simulink model "teste_bar_dados_5_1"  (R2020a)
settings: Solver=VariableStepAuto  StartTime=0.0  StopTime=10.0  RelTol=1e-3
values from neighbouring files (symbols this model uses):
  sample_time = 0.03    [lab3.m]
settings Model: Creator=josem  LastModifiedBy=josem

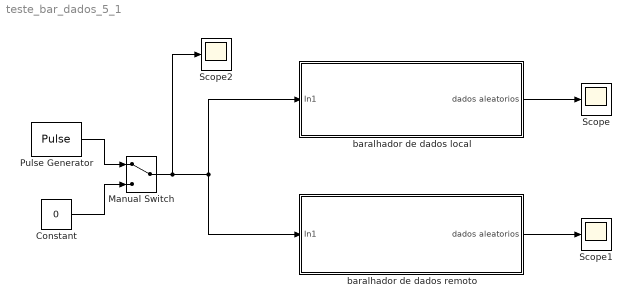
== system teste_bar_dados_5_1 ==
  Constant : Constant  Value=0  SampleTime=sample_time
  Manual Switch : ManualSwitch
  Pulse Generator : DiscretePulseGenerator  Period=10  PulseWidth=5  SampleTime=sample_time
  Scope : Scope
  Scope1 : Scope
  Scope2 : Scope
  baralhador de dados local : Subsystem
  baralhador de dados remoto : Subsystem
  wires:
  Manual Switch/1 -> Scope2/1, baralhador de dados local/1(In1), baralhador de dados remoto/1(In1)
  Pulse Generator/1 -> Manual Switch/1
  Constant/1 -> Manual Switch/2
  baralhador de dados local/1(dados aleatorios) -> Scope/1
  baralhador de dados remoto/1(dados aleatorios) -> Scope1/1

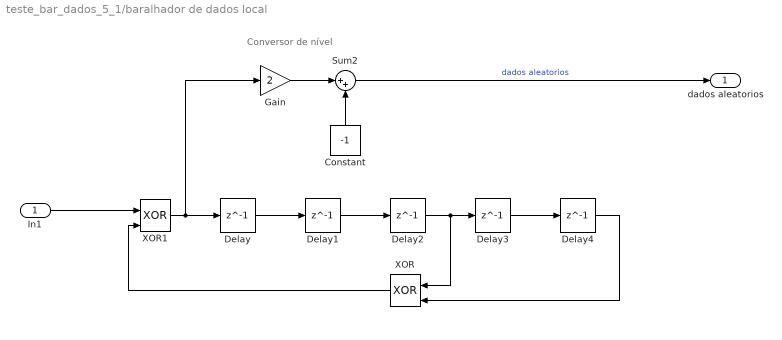
== system teste_bar_dados_5_1/baralhador de dados local ==
  note: Conversor de nível
  In1 : Inport
  Constant : Constant  Value=-1
  Delay{,1..4} (5 alike) : Delay  DelayLength=1  InitialCondition=0
  Gain : Gain  Gain=2
  Sum2 : Sum  Inputs=|++
  XOR : Logic  Operator=XOR  IconShape=distinctive  AllPortsSameDT=off  OutDataTypeStr=boolean
  XOR1 : Logic  Operator=XOR  IconShape=distinctive  AllPortsSameDT=off  OutDataTypeStr=boolean
  dados aleatorios : Outport
  wires:
  Delay4/1 -> XOR/2
  XOR1/1 -> Gain/1, Delay/1
  Constant/1 -> Sum2/2
  Delay/1 -> Delay1/1
  Delay2/1 -> XOR/1, Delay3/1
  Gain/1 -> Sum2/1
  XOR/1 -> XOR1/2
  Delay3/1 -> Delay4/1
  Delay1/1 -> Delay2/1
  Sum2/1 -> dados aleatorios/1  "dados aleatorios"
  In1/1 -> XOR1/1

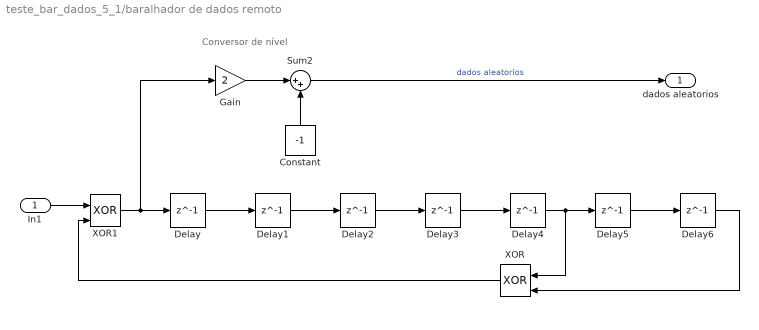
== system teste_bar_dados_5_1/baralhador de dados remoto ==
  note: Conversor de nível
  In1 : Inport
  Constant : Constant  Value=-1
  Delay{,1..6} (7 alike) : Delay  DelayLength=1  InitialCondition=0
  Gain : Gain  Gain=2
  Sum2 : Sum  Inputs=|++
  XOR : Logic  Operator=XOR  IconShape=distinctive  AllPortsSameDT=off  OutDataTypeStr=boolean
  XOR1 : Logic  Operator=XOR  IconShape=distinctive  AllPortsSameDT=off  OutDataTypeStr=boolean
  dados aleatorios : Outport
  wires:
  XOR/1 -> XOR1/2
  Delay1/1 -> Delay2/1
  Delay3/1 -> Delay4/1
  XOR1/1 -> Gain/1, Delay/1
  Delay/1 -> Delay1/1
  Delay5/1 -> Delay6/1
  Sum2/1 -> dados aleatorios/1  "dados aleatorios"
  Delay4/1 -> XOR/1, Delay5/1
  Gain/1 -> Sum2/1
  Delay6/1 -> XOR/2
  Delay2/1 -> Delay3/1
  Constant/1 -> Sum2/2
  In1/1 -> XOR1/1
